simulink model "BPSK_Modulation"  (R2013a)
settings: Solver=VariableStepDiscrete  StartTime=0.0  StopTime=0.2  RelTol=1e-3
libraries: simulink_extras x4, dsparch4 x2, dspspect3 x1, commrandsrc2 x1
settings Model: Creator=Cedric  LastModifiedBy=Cedric
settings OptimizationCC: BooleanDataType=off

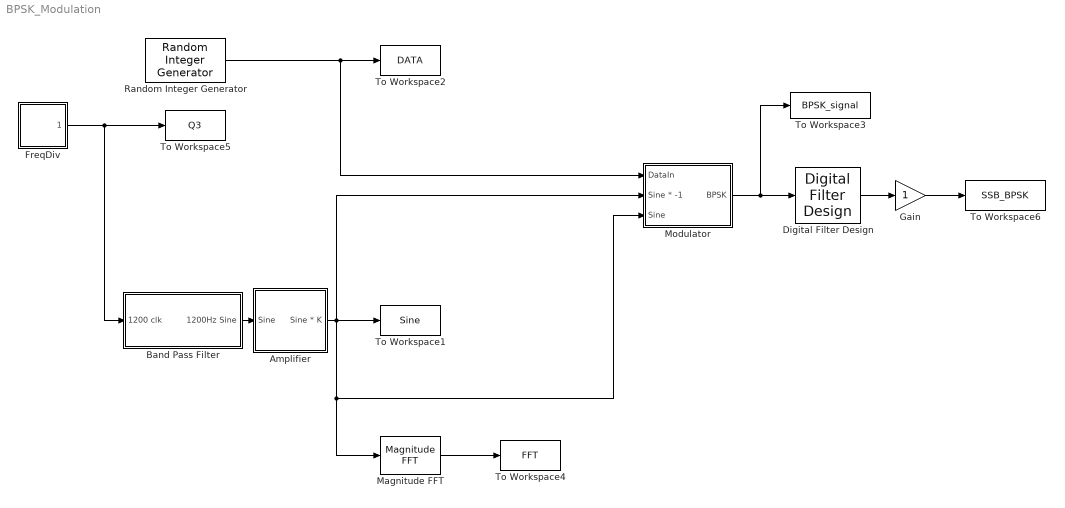
== system BPSK_Modulation ==
  Amplifier : Subsystem
  Band Pass Filter : Subsystem
  Digital Filter Design : dsparch4/Digital Filter Design  mwdsp_browser_bugfix_var=off
  FreqDiv : Subsystem
  Gain : Gain
  Magnitude FFT : dspspect3/Magnitude FFT  mag_or_magsq=Magnitude squared  FFTImplementation=Auto  fftLenInherit=off  fftsize=256
  Modulator : Subsystem
  Random Integer Generator : commrandsrc2/Random Integer Generator  mul=2  seed=randseed  Ts=1/600  frameBased=off  sampPerFrame=1  orient=on  outDataType=double
  To Workspace1 : ToWorkspace  VariableName=Sine  SampleTime=5e-6  SaveFormat=Timeseries
  To Workspace2 : ToWorkspace  VariableName=DATA  SampleTime=5e-6  SaveFormat=Timeseries
  To Workspace3 : ToWorkspace  VariableName=BPSK_signal  SampleTime=5e-6  SaveFormat=Timeseries
  To Workspace4 : ToWorkspace  VariableName=FFT  SampleTime=5e-6  SaveFormat=Timeseries
  To Workspace5 : ToWorkspace  VariableName=Q3  SampleTime=-1  SaveFormat=Timeseries
  To Workspace6 : ToWorkspace  VariableName=SSB_BPSK  SampleTime=5e-6  SaveFormat=Timeseries
  wires:
  FreqDiv/1("1200Clk ") -> Band Pass Filter/1(1200 clk), To Workspace5/1
  Random Integer Generator/1 -> Modulator/1(DataIn), To Workspace2/1
  Amplifier/1(Sine * K) -> Modulator/2(Sine * -1), Magnitude FFT/1, Modulator/3(Sine), To Workspace1/1
  Band Pass Filter/1(1200Hz Sine) -> Amplifier/1(Sine)
  Modulator/1(BPSK) -> Digital Filter Design/1, To Workspace3/1
  Magnitude FFT/1 -> To Workspace4/1
  Digital Filter Design/1 -> Gain/1
  Gain/1 -> To Workspace6/1

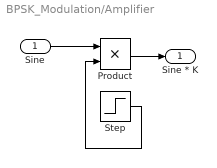
== system BPSK_Modulation/Amplifier ==
  Sine : Inport
  Product : Product
  Step : Step  Time=0.0150  SampleTime=5e-6
  Sine * K : Outport
  wires:
  Sine/1 -> Product/1
  Step/1 -> Product/2
  Product/1 -> Sine * K/1

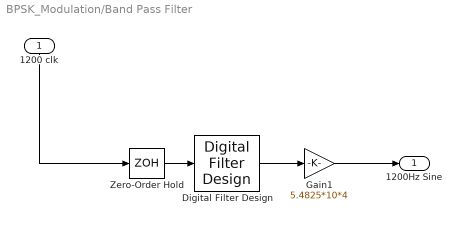
== system BPSK_Modulation/Band Pass Filter ==
  1200 clk : Inport
  Digital Filter Design : dsparch4/Digital Filter Design  mwdsp_browser_bugfix_var=off
  Gain1 : Gain  Gain=5.4825*10*4
  Zero-Order Hold : ZeroOrderHold  SampleTime=5e-6
  1200Hz Sine : Outport
  wires:
  Zero-Order Hold/1 -> Digital Filter Design/1
  Digital Filter Design/1 -> Gain1/1
  1200 clk/1 -> Zero-Order Hold/1
  Gain1/1 -> 1200Hz Sine/1

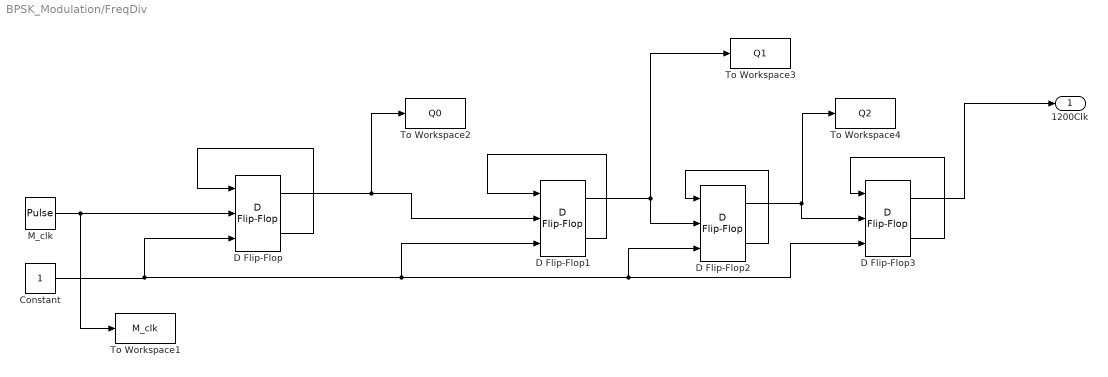
== system BPSK_Modulation/FreqDiv ==
  Constant : Constant
  D Flip-Flop{,1..3} (4 alike) : simulink_extras/Flip Flops/D Flip-Flop
  M_clk : DiscretePulseGenerator  PulseType=Time based  Period=1/19200  PulseWidth=50
  To Workspace1 : ToWorkspace  VariableName=M_clk  SampleTime=5e-6  SaveFormat=Timeseries
  To Workspace2 : ToWorkspace  VariableName=Q0  SampleTime=-1  SaveFormat=Timeseries
  To Workspace3 : ToWorkspace  VariableName=Q1  SampleTime=-1  SaveFormat=Timeseries
  To Workspace4 : ToWorkspace  VariableName=Q2  SampleTime=-1  SaveFormat=Timeseries
  "1200Clk " : Outport
  wires:
  D Flip-Flop/1 -> To Workspace2/1, D Flip-Flop1/2
  M_clk/1 -> To Workspace1/1, D Flip-Flop/2
  D Flip-Flop3/2 -> D Flip-Flop3/1
  Constant/1 -> D Flip-Flop3/3, D Flip-Flop2/3, D Flip-Flop1/3, D Flip-Flop/3
  D Flip-Flop2/1 -> D Flip-Flop3/2, To Workspace4/1
  D Flip-Flop1/1 -> To Workspace3/1, D Flip-Flop2/2
  D Flip-Flop2/2 -> D Flip-Flop2/1
  D Flip-Flop/2 -> D Flip-Flop/1
  D Flip-Flop1/2 -> D Flip-Flop1/1
  D Flip-Flop3/1 -> "1200Clk "/1

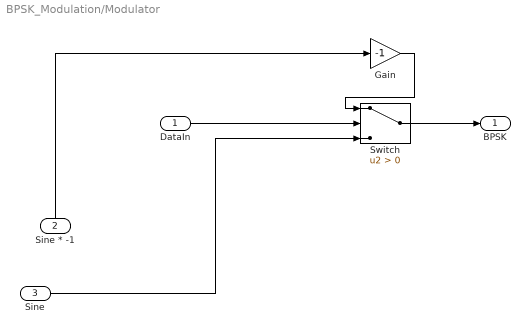
== system BPSK_Modulation/Modulator ==
  DataIn : Inport
  Sine * -1 : Inport  Port=2
  Sine : Inport  Port=3
  Gain : Gain  Gain=-1
  Switch : Switch  Criteria=u2 > Threshold  SampleTime=5e-6
  BPSK : Outport
  wires:
  DataIn/1 -> Switch/2
  Sine/1 -> Switch/3
  Sine * -1/1 -> Gain/1
  Gain/1 -> Switch/1
  Switch/1 -> BPSK/1
